simulink model "sim_nomal_regulator"  (R2019a)
settings: Solver=FixedStepAuto  StartTime=0.0  StopTime=20  FixedStep=sT  RelTol=1e-3
InitFcn:
  | sim_param;
values from neighbouring files (symbols this model uses):
  bn = 50    [robot_param.m]    (also in sim_robot_param.m)
  bt = 50    [robot_param.m]    (also in sim_robot_param.m)
  foot_x = 0.07    [robot_param.m]    (also in sim_robot_param.m)
  foot_y = 0.045    [robot_param.m]    (also in sim_robot_param.m)
  foot_z = 0.01    [robot_param.m]    (also in sim_robot_param.m)
  height_plane = 0.025    [robot_param.m]    (also in sim_robot_param.m)
  inix = [0.00 0.00]'    [param.m]    (also in sim_param.m)
  iniXzmax = 0.05    [param.m]    (also in sim_param.m)
  iniXzmin = -0.05    [param.m]    (also in sim_param.m)
  iniy = [0.00 0.00]'    [param.m]    (also in sim_param.m)
  iniYzmax = 0.0625    [param.m]    (also in sim_param.m)
  iniYzmin = -0.0625    [param.m]    (also in sim_param.m)
  kn = 5000    [robot_param.m]    (also in sim_robot_param.m)
  kt = 5000    [robot_param.m]    (also in sim_robot_param.m)
  mu_d = 0.8    [robot_param.m]    (also in sim_robot_param.m)
  mu_s = 2    [robot_param.m]    (also in sim_robot_param.m)
  plane_x = 3    [robot_param.m]    (also in sim_robot_param.m = 6)
  plane_y = 1    [robot_param.m]    (also in sim_robot_param.m)
  R = 20    [param.m]    (also in sim_param.m = 1)
  sT = 0.02    [param.m]    (also in sim_param.m = 0.001)
  torso_offset_x = 0.0    (= 0)    [robot_param.m]    (also in sim_robot_param.m)
  torso_offset_z = -torso_z/2    (= -0.05)    [robot_param.m]    (also in sim_robot_param.m)
  torso_x = 0.1    [robot_param.m]    (also in sim_robot_param.m)
  torso_y = 0.08    [robot_param.m]    (also in sim_robot_param.m)
  torso_z = 0.10    (= 0.1)    [robot_param.m]    (also in sim_robot_param.m)
  w = sqrt(g/zc)    [param.m]    (also in sim_param.m)
  zvt = 1e-3    (= 0.001)    [robot_param.m]    (also in sim_robot_param.m)
undefined symbols (not defined in the file or in its folder): Ad, Bd, Cd, Dd, DiscIntNeverNeededParam, Discrete, sigbuilder_block, Time, X, Y, Z
libraries: nesl_utility x142, sm_lib x86, cstblocks x11, ctrlSharedLib x8
(part 1 of 6)
settings Model: Creator=hideaki  LastModifiedBy=hideaki

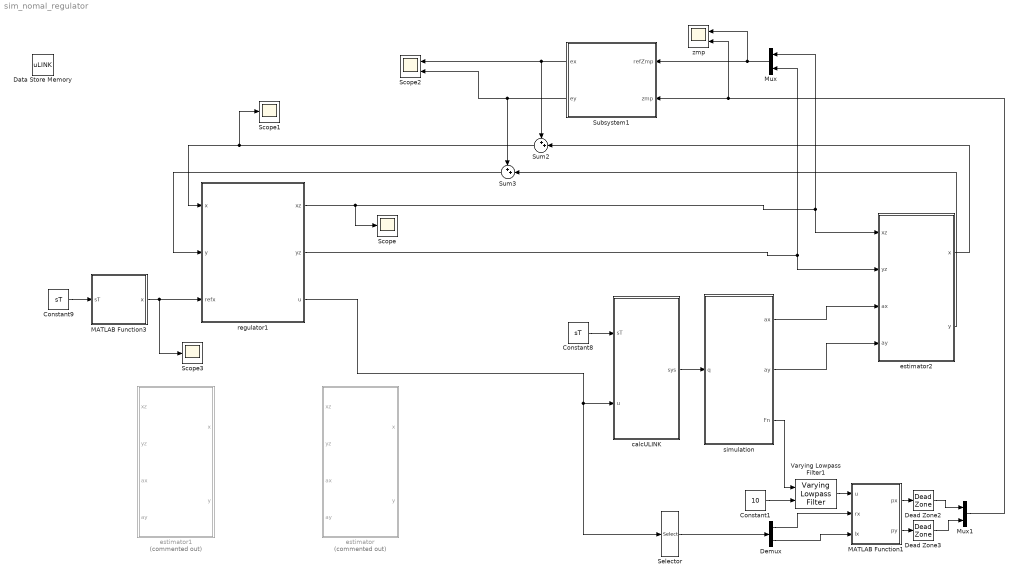
== system sim_nomal_regulator ==
  Constant1 : Constant  Value=10
  Constant8 : Constant  Value=sT
  Constant9 : Constant  Value=sT
  Data Store Memory : DataStoreMemory  DataStoreName=uLINK  ReadBeforeWriteMsg=warning  WriteAfterWriteMsg=warning  WriteAfterReadMsg=warning  InitialValue=uLINK  ShowAdditionalParam=off  OutDataTypeStr=Bus: ULINK  Dimensions=[15 1]
  Dead Zone2 : DeadZone  LowerValue=-1e-5  UpperValue=1e-5  SaturateOnIntegerOverflow=on
  Dead Zone3 : DeadZone  LowerValue=-1e-5  UpperValue=1e-5  SaturateOnIntegerOverflow=on
  Demux : Demux  Outputs=2
  MATLAB Function1 : MATLAB Function  TreatAsAtomicUnit=on
  MATLAB Function3 : MATLAB Function  TreatAsAtomicUnit=on  SystemSampleTime=sT
  Mux : Mux  Inputs=2
  Mux1 : Mux  Inputs=2
  Scope : Scope
  Scope1 : Scope
  Scope2 : Scope  NumInputPorts=2
  Scope3 : Scope
  Selector : Selector  InputPortWidth=8  IndexOptions=Index vector (dialog)  Indices=[3 6]  OutputSizes=1
  Subsystem1 : Subsystem
  Sum2 : Sum  Inputs=++|
  Sum3 : Sum  Inputs=++|
  Varying Lowpass Filter1 : cstblocks/Linear Parameter Varying/Varying Lowpass Filter  N=1
      settings: SourceProductName=Control System Toolbox
  calcULINK : MATLAB Function  TreatAsAtomicUnit=on
  estimator : Subsystem  Commented=on
  estimator1 : Subsystem  Commented=on
  estimator2 : Subsystem
  regulator1 : Subsystem
  simulation : Subsystem
  zmp : Scope  NumInputPorts=2
  wires:
  Constant8/1 -> calcULINK/1(sT)
  calcULINK/1(sys) -> simulation/1(q)
  Constant9/1 -> MATLAB Function3/1(sT)
  simulation/1(ax) -> estimator2/3(ax)
  simulation/2(ay) -> estimator2/4(ay)
  estimator2/2(y) -> Sum3/2
  MATLAB Function3/1(x) -> Scope3/1, regulator1/3(refx)
  regulator1/1(xz) -> Scope/1, estimator2/1(xz), Mux/1
  regulator1/2(yz) -> estimator2/2(yz), Mux/2
  estimator2/1(x) -> Sum2/2
  Varying Lowpass Filter1/1 -> MATLAB Function1/1(u)
  Constant1/1 -> Varying Lowpass Filter1/2
  MATLAB Function1/1(px) -> Dead Zone2/1
  Selector/1 -> Demux/1
  simulation/3(Fn) -> Varying Lowpass Filter1/1
  Demux/1 -> MATLAB Function1/2(rx)
  regulator1/3(u) -> Selector/1, calcULINK/2(u)
  Demux/2 -> MATLAB Function1/3(lx)
  MATLAB Function1/2(py) -> Dead Zone3/1
  Dead Zone2/1 -> Mux1/1
  Dead Zone3/1 -> Mux1/2
  Mux/1 -> zmp/1, Subsystem1/1(refZmp)
  Mux1/1 -> zmp/2, Subsystem1/2(zmp)
  Subsystem1/1(ex) -> Sum2/1, Scope2/1
  Subsystem1/2(ey) -> Sum3/1, Scope2/2
  Sum3/1 -> regulator1/2(y)
  Sum2/1 -> Scope1/1, regulator1/1(x)

== system sim_nomal_regulator/Subsystem1 ==
  note: alphaを外すとおかしくなる
  refZmp : Inport
  zmp : Inport  Port=2
  Demux : Demux  Outputs=2
  Demux2 : Demux  Outputs=2
  Discrete-Time Integrator : DiscreteIntegrator  gainval=1.6  SampleTime=-1  ICPrevOutput=DiscIntNeverNeededParam  ICPrevScaledInput=DiscIntNeverNeededParam
  Discrete-Time Integrator1 : DiscreteIntegrator  SampleTime=-1  ICPrevOutput=DiscIntNeverNeededParam  ICPrevScaledInput=DiscIntNeverNeededParam
  Discrete-Time Integrator2 : DiscreteIntegrator  gainval=1.6  SampleTime=-1  ICPrevOutput=DiscIntNeverNeededParam  ICPrevScaledInput=DiscIntNeverNeededParam
  Discrete-Time Integrator3 : DiscreteIntegrator  SampleTime=-1  ICPrevOutput=DiscIntNeverNeededParam  ICPrevScaledInput=DiscIntNeverNeededParam
  Gain2 : Gain  Gain=0.1
  Gain4 : Gain  Gain=25
  Mux3 : Mux  Inputs=2
  Mux4 : Mux  Inputs=2
  Sum : Sum  Inputs=|-+
  Sum1 : Sum  Inputs=|-+
  Sum3 : Sum  Inputs=+-|
  Sum4 : Sum  Inputs=+-|
  alphax : Constant  Value=0
  alphay : Constant  Value=0
  ex : Outport
  ey : Outport  Port=2
  wires:
  Gain4/1 -> Sum/1
  Demux2/1 -> Sum3/1
  Discrete-Time Integrator2/1 -> Discrete-Time Integrator3/1, Mux4/2
  Demux/1 -> Sum3/2
  Discrete-Time Integrator3/1 -> Mux4/1
  Mux3/1 -> ex/1
  Discrete-Time Integrator1/1 -> Mux3/1
  Demux2/2 -> Sum4/1
  Gain2/1 -> Sum1/1
  Discrete-Time Integrator/1 -> Mux3/2, Discrete-Time Integrator1/1
  Mux4/1 -> ey/1
  Demux/2 -> Sum4/2
  Sum3/1 -> Gain2/1
  zmp/1 -> Demux/1
  Sum4/1 -> Gain4/1
  refZmp/1 -> Demux2/1
  Sum/1 -> Discrete-Time Integrator2/1
  alphay/1 -> Sum/2
  alphax/1 -> Sum1/2
  Sum1/1 -> Discrete-Time Integrator/1

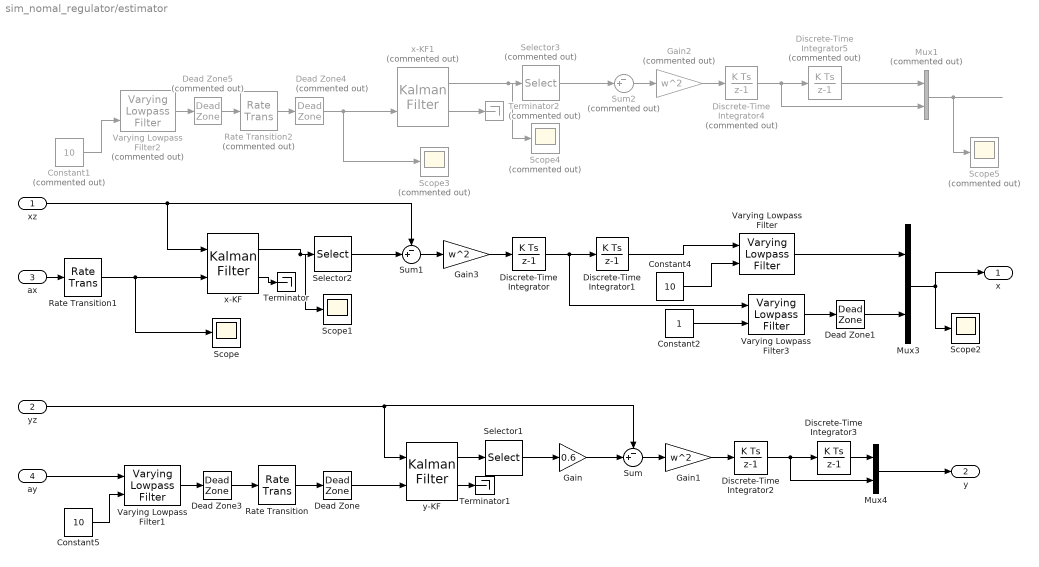
== system sim_nomal_regulator/estimator ==
  xz : Inport
  yz : Inport  Port=2
  ax : Inport  Port=3
  ay : Inport  Port=4
  Constant1 : Constant  Commented=on  Value=10
  Constant2 : Constant
  Constant4 : Constant  Value=10
  Constant5 : Constant  Value=10
  Dead Zone : DeadZone  LowerValue=-1e-3  UpperValue=1e-3  SaturateOnIntegerOverflow=on
  Dead Zone1 : DeadZone  LowerValue=-5e-2  UpperValue=5e-2  SaturateOnIntegerOverflow=on
  Dead Zone3 : DeadZone  LowerValue=-5e-2  UpperValue=5e-2  SaturateOnIntegerOverflow=on
  Dead Zone4 : DeadZone  Commented=on  LowerValue=-1e-3  UpperValue=1e-3  SaturateOnIntegerOverflow=on
  Dead Zone5 : DeadZone  Commented=on  LowerValue=-5e-2  UpperValue=5e-2  SaturateOnIntegerOverflow=on
  Discrete-Time Integrator : DiscreteIntegrator  gainval=1.6  SampleTime=-1  ICPrevOutput=DiscIntNeverNeededParam  ICPrevScaledInput=DiscIntNeverNeededParam
  Discrete-Time Integrator1 : DiscreteIntegrator  SampleTime=-1  ICPrevOutput=DiscIntNeverNeededParam  ICPrevScaledInput=DiscIntNeverNeededParam
  Discrete-Time Integrator2 : DiscreteIntegrator  SampleTime=-1  ICPrevOutput=DiscIntNeverNeededParam  ICPrevScaledInput=DiscIntNeverNeededParam
  Discrete-Time Integrator3 : DiscreteIntegrator  SampleTime=-1  ICPrevOutput=DiscIntNeverNeededParam  ICPrevScaledInput=DiscIntNeverNeededParam
  Discrete-Time Integrator4 : DiscreteIntegrator  Commented=on  gainval=1.6  SampleTime=-1  ICPrevOutput=DiscIntNeverNeededParam  ICPrevScaledInput=DiscIntNeverNeededParam
  Discrete-Time Integrator5 : DiscreteIntegrator  Commented=on  SampleTime=-1  ICPrevOutput=DiscIntNeverNeededParam  ICPrevScaledInput=DiscIntNeverNeededParam
  Gain : Gain  Gain=0.6
  Gain1 : Gain  Gain=w^2
  Gain2 : Gain  Commented=on  Gain=w^2
  Gain3 : Gain  Gain=w^2
  Mux1 : Mux  Commented=on  Inputs=2
  Mux3 : Mux  Inputs=2
  Mux4 : Mux  Inputs=2
  Rate Transition : RateTransition  OutPortSampleTime=sT
  Rate Transition1 : RateTransition  OutPortSampleTime=sT
  Rate Transition2 : RateTransition  Commented=on  OutPortSampleTime=sT
  Scope : Scope
  Scope1 : Scope
  Scope2 : Scope
  Scope3 : Scope  Commented=on
  Scope4 : Scope  Commented=on
  Scope5 : Scope  Commented=on
  Selector1 : Selector  InputPortWidth=2  IndexOptions=Index vector (dialog)  Indices=[1]  OutputSizes=1
  Selector2 : Selector  InputPortWidth=2  IndexOptions=Index vector (dialog)  Indices=[1]  OutputSizes=1
  Selector3 : Selector  Commented=on  InputPortWidth=2  IndexOptions=Index vector (dialog)  Indices=[1]  OutputSizes=1
  Sum : Sum  Inputs=-+|
  Sum1 : Sum  Inputs=-+|
  Sum2 : Sum  Commented=on  Inputs=-+|
  Terminator : Terminator
  Terminator1 : Terminator
  Terminator2 : Terminator  Commented=on
  Varying Lowpass Filter : cstblocks/Linear Parameter Varying/Varying Lowpass Filter  N=1
      settings: SourceProductName=Control System Toolbox
  Varying Lowpass Filter1 : cstblocks/Linear Parameter Varying/Varying Lowpass Filter  N=1
      settings: SourceProductName=Control System Toolbox
  Varying Lowpass Filter2 : cstblocks/Linear Parameter Varying/Varying Lowpass Filter  Commented=on  N=1
      settings: SourceProductName=Control System Toolbox
  Varying Lowpass Filter3 : cstblocks/Linear Parameter Varying/Varying Lowpass Filter  N=1
      settings: SourceProductName=Control System Toolbox
  x-KF : ctrlSharedLib/Kalman Filter  TimeDomain=Discrete-Time  UseCurrentEstimator=on  ModelSource=Individual A, B, C, D matrices  ModelSourceVariable=ss(0.95,1,1,0,1)  A=Ad  B=Bd  C=Cd  D=Dd  NumberOfStates=1  NumberOfInputs=1  NumberOfOutputs=1  InitialEstimateSource=Dialog  X0=inix  P0=[100 50]'  UseK=off  UseGH=off  NumberOfProcessNoiseInputs=1  G=[0 0]'  TimeInvariantG=on  H=10  TimeInvariantH=on  Q=Q  TimeInvariantQ=on  R=R  TimeInvariantR=on  N=0  TimeInvariantN=on  AddInputPort=on  AddEnablePort=off  OutputEstimatedY=on  OutputP=off  Ts=sT
      settings: SourceProductBaseCode=CT
  x-KF1 : ctrlSharedLib/Kalman Filter  Commented=on  TimeDomain=Discrete-Time  UseCurrentEstimator=on  ModelSource=Individual A, B, C, D matrices  ModelSourceVariable=ss(0.95,1,1,0,1)  A=Ad  B=Bd  C=Cd  D=Dd  NumberOfStates=1  NumberOfInputs=1  NumberOfOutputs=1  InitialEstimateSource=Dialog  X0=inix  P0=[100 50]'  UseK=off  UseGH=off  NumberOfProcessNoiseInputs=1  G=[0 0]'  TimeInvariantG=on  H=10  TimeInvariantH=on  Q=Q  TimeInvariantQ=on  R=R  TimeInvariantR=on  N=0  TimeInvariantN=on  AddInputPort=on  AddEnablePort=off  OutputEstimatedY=on  OutputP=off  Ts=sT
      settings: SourceProductBaseCode=CT
  y-KF : ctrlSharedLib/Kalman Filter  TimeDomain=Discrete-Time  UseCurrentEstimator=on  ModelSource=Individual A, B, C, D matrices  ModelSourceVariable=ss(0.95,1,1,0,1)  A=Ad  B=Bd  C=Cd  D=Dd  NumberOfStates=1  NumberOfInputs=1  NumberOfOutputs=1  InitialEstimateSource=Dialog  X0=iniy  P0=10  UseK=off  UseGH=off  NumberOfProcessNoiseInputs=1  G=[0 0]'  TimeInvariantG=on  H=10  TimeInvariantH=on  Q=Q  TimeInvariantQ=on  R=R  TimeInvariantR=on  N=0  TimeInvariantN=on  AddInputPort=on  AddEnablePort=off  OutputEstimatedY=on  OutputP=off  Ts=sT
      settings: SourceProductBaseCode=CT
  x : Outport
  y : Outport  Port=2
  wires:
  Sum/1 -> Gain1/1
  Dead Zone/1 -> y-KF/2
  Selector1/1 -> Gain/1
  Discrete-Time Integrator2/1 -> Discrete-Time Integrator3/1, Mux4/2
  Sum1/1 -> Gain3/1
  Discrete-Time Integrator3/1 -> Mux4/1
  Discrete-Time Integrator/1 -> Varying Lowpass Filter3/1, Discrete-Time Integrator1/1
  Gain3/1 -> Discrete-Time Integrator/1
  y-KF/2 -> Terminator1/1
  Gain1/1 -> Discrete-Time Integrator2/1
  Varying Lowpass Filter1/1 -> Dead Zone3/1
  xz/1 -> Sum1/1, x-KF/1
  Rate Transition/1 -> Dead Zone/1
  y-KF/1 -> Selector1/1
  Constant4/1 -> Varying Lowpass Filter/2
  Constant5/1 -> Varying Lowpass Filter1/2
  Varying Lowpass Filter/1 -> Mux3/1
  x-KF/1 -> Scope1/1, Selector2/1
  yz/1 -> y-KF/1, Sum/1
  Discrete-Time Integrator1/1 -> Varying Lowpass Filter/1
  Gain/1 -> Sum/2
  Selector2/1 -> Sum1/2
  Mux3/1 -> Scope2/1, x/1
  Mux4/1 -> y/1
  x-KF/2 -> Terminator/1
  ay/1 -> Varying Lowpass Filter1/1
  ax/1 -> Rate Transition1/1
  Dead Zone3/1 -> Rate Transition/1
  Dead Zone5/1 -> Rate Transition2/1
  Dead Zone4/1 -> Scope3/1, x-KF1/2
  Rate Transition2/1 -> Dead Zone4/1
  x-KF1/2 -> Terminator2/1
  Selector3/1 -> Sum2/2
  Mux1/1 -> Scope5/1
  x-KF1/1 -> Scope4/1, Selector3/1
  Constant1/1 -> Varying Lowpass Filter2/2
  ? -> Varying Lowpass Filter2/1
  Gain2/1 -> Discrete-Time Integrator4/1
  Discrete-Time Integrator5/1 -> Mux1/1
  ? -> Sum2/1, x-KF1/1
  Varying Lowpass Filter2/1 -> Dead Zone5/1
  Discrete-Time Integrator4/1 -> Discrete-Time Integrator5/1, Mux1/2
  Sum2/1 -> Gain2/1
  Varying Lowpass Filter3/1 -> Dead Zone1/1
  Rate Transition1/1 -> Scope/1, x-KF/2
  Constant2/1 -> Varying Lowpass Filter3/2
  Dead Zone1/1 -> Mux3/2

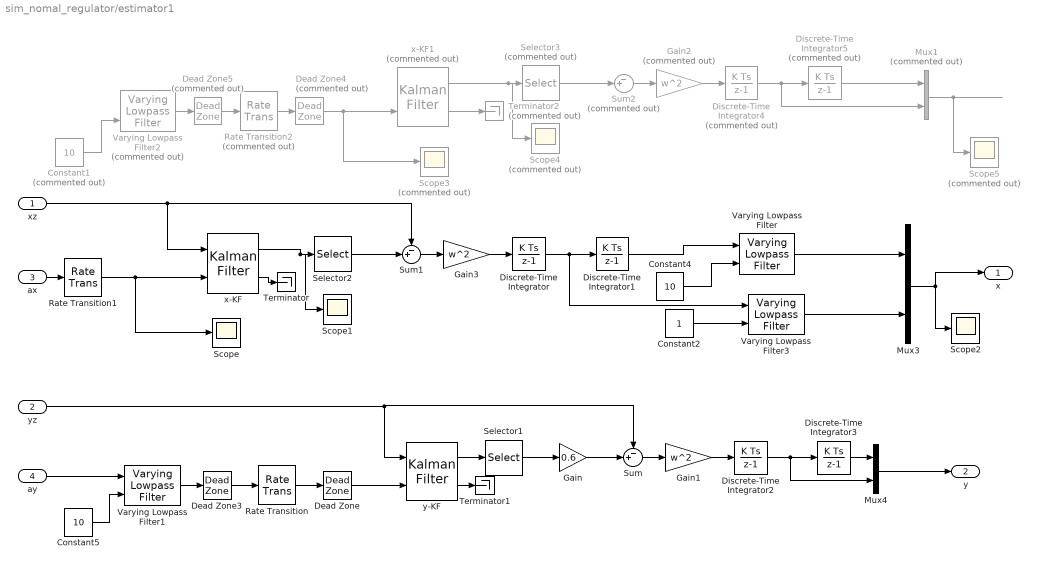
== system sim_nomal_regulator/estimator1 ==
  xz : Inport
  yz : Inport  Port=2
  ax : Inport  Port=3
  ay : Inport  Port=4
  Constant1 : Constant  Commented=on  Value=10
  Constant2 : Constant
  Constant4 : Constant  Value=10
  Constant5 : Constant  Value=10
  Dead Zone : DeadZone  LowerValue=-1e-3  UpperValue=1e-3  SaturateOnIntegerOverflow=on
  Dead Zone3 : DeadZone  LowerValue=-5e-2  UpperValue=5e-2  SaturateOnIntegerOverflow=on
  Dead Zone4 : DeadZone  Commented=on  LowerValue=-1e-3  UpperValue=1e-3  SaturateOnIntegerOverflow=on
  Dead Zone5 : DeadZone  Commented=on  LowerValue=-5e-2  UpperValue=5e-2  SaturateOnIntegerOverflow=on
  Discrete-Time Integrator : DiscreteIntegrator  gainval=1.6  SampleTime=-1  ICPrevOutput=DiscIntNeverNeededParam  ICPrevScaledInput=DiscIntNeverNeededParam
  Discrete-Time Integrator1 : DiscreteIntegrator  SampleTime=-1  ICPrevOutput=DiscIntNeverNeededParam  ICPrevScaledInput=DiscIntNeverNeededParam
  Discrete-Time Integrator2 : DiscreteIntegrator  SampleTime=-1  ICPrevOutput=DiscIntNeverNeededParam  ICPrevScaledInput=DiscIntNeverNeededParam
  Discrete-Time Integrator3 : DiscreteIntegrator  SampleTime=-1  ICPrevOutput=DiscIntNeverNeededParam  ICPrevScaledInput=DiscIntNeverNeededParam
  Discrete-Time Integrator4 : DiscreteIntegrator  Commented=on  gainval=1.6  SampleTime=-1  ICPrevOutput=DiscIntNeverNeededParam  ICPrevScaledInput=DiscIntNeverNeededParam
  Discrete-Time Integrator5 : DiscreteIntegrator  Commented=on  SampleTime=-1  ICPrevOutput=DiscIntNeverNeededParam  ICPrevScaledInput=DiscIntNeverNeededParam
  Gain : Gain  Gain=0.6
  Gain1 : Gain  Gain=w^2
  Gain2 : Gain  Commented=on  Gain=w^2
  Gain3 : Gain  Gain=w^2
  Mux1 : Mux  Commented=on  Inputs=2
  Mux3 : Mux  Inputs=2
  Mux4 : Mux  Inputs=2
  Rate Transition : RateTransition  OutPortSampleTime=sT
  Rate Transition1 : RateTransition  OutPortSampleTime=sT
  Rate Transition2 : RateTransition  Commented=on  OutPortSampleTime=sT
  Scope : Scope
  Scope1 : Scope
  Scope2 : Scope
  Scope3 : Scope  Commented=on
  Scope4 : Scope  Commented=on
  Scope5 : Scope  Commented=on
  Selector1 : Selector  InputPortWidth=2  IndexOptions=Index vector (dialog)  Indices=[1]  OutputSizes=1
  Selector2 : Selector  InputPortWidth=2  IndexOptions=Index vector (dialog)  Indices=[1]  OutputSizes=1
  Selector3 : Selector  Commented=on  InputPortWidth=2  IndexOptions=Index vector (dialog)  Indices=[1]  OutputSizes=1
  Sum : Sum  Inputs=-+|
  Sum1 : Sum  Inputs=-+|
  Sum2 : Sum  Commented=on  Inputs=-+|
  Terminator : Terminator
  Terminator1 : Terminator
  Terminator2 : Terminator  Commented=on
  Varying Lowpass Filter : cstblocks/Linear Parameter Varying/Varying Lowpass Filter  N=1
      settings: SourceProductName=Control System Toolbox
  Varying Lowpass Filter1 : cstblocks/Linear Parameter Varying/Varying Lowpass Filter  N=1
      settings: SourceProductName=Control System Toolbox
  Varying Lowpass Filter2 : cstblocks/Linear Parameter Varying/Varying Lowpass Filter  Commented=on  N=1
      settings: SourceProductName=Control System Toolbox
  Varying Lowpass Filter3 : cstblocks/Linear Parameter Varying/Varying Lowpass Filter  N=1
      settings: SourceProductName=Control System Toolbox
  x-KF : ctrlSharedLib/Kalman Filter  TimeDomain=Discrete-Time  UseCurrentEstimator=on  ModelSource=Individual A, B, C, D matrices  ModelSourceVariable=ss(0.95,1,1,0,1)  A=Ad  B=Bd  C=Cd  D=Dd  NumberOfStates=1  NumberOfInputs=1  NumberOfOutputs=1  InitialEstimateSource=Dialog  X0=inix  P0=[100 50]'  UseK=off  UseGH=off  NumberOfProcessNoiseInputs=1  G=[0 0]'  TimeInvariantG=on  H=10  TimeInvariantH=on  Q=Q  TimeInvariantQ=on  R=R  TimeInvariantR=on  N=0  TimeInvariantN=on  AddInputPort=on  AddEnablePort=off  OutputEstimatedY=on  OutputP=off  Ts=sT
      settings: SourceProductBaseCode=CT
  x-KF1 : ctrlSharedLib/Kalman Filter  Commented=on  TimeDomain=Discrete-Time  UseCurrentEstimator=on  ModelSource=Individual A, B, C, D matrices  ModelSourceVariable=ss(0.95,1,1,0,1)  A=Ad  B=Bd  C=Cd  D=Dd  NumberOfStates=1  NumberOfInputs=1  NumberOfOutputs=1  InitialEstimateSource=Dialog  X0=inix  P0=[100 50]'  UseK=off  UseGH=off  NumberOfProcessNoiseInputs=1  G=[0 0]'  TimeInvariantG=on  H=10  TimeInvariantH=on  Q=Q  TimeInvariantQ=on  R=R  TimeInvariantR=on  N=0  TimeInvariantN=on  AddInputPort=on  AddEnablePort=off  OutputEstimatedY=on  OutputP=off  Ts=sT
      settings: SourceProductBaseCode=CT
  y-KF : ctrlSharedLib/Kalman Filter  TimeDomain=Discrete-Time  UseCurrentEstimator=on  ModelSource=Individual A, B, C, D matrices  ModelSourceVariable=ss(0.95,1,1,0,1)  A=Ad  B=Bd  C=Cd  D=Dd  NumberOfStates=1  NumberOfInputs=1  NumberOfOutputs=1  InitialEstimateSource=Dialog  X0=iniy  P0=10  UseK=off  UseGH=off  NumberOfProcessNoiseInputs=1  G=[0 0]'  TimeInvariantG=on  H=10  TimeInvariantH=on  Q=Q  TimeInvariantQ=on  R=R  TimeInvariantR=on  N=0  TimeInvariantN=on  AddInputPort=on  AddEnablePort=off  OutputEstimatedY=on  OutputP=off  Ts=sT
      settings: SourceProductBaseCode=CT
  x : Outport
  y : Outport  Port=2
  wires:
  Sum/1 -> Gain1/1
  Dead Zone/1 -> y-KF/2
  Selector1/1 -> Gain/1
  Discrete-Time Integrator2/1 -> Discrete-Time Integrator3/1, Mux4/2
  Sum1/1 -> Gain3/1
  Discrete-Time Integrator3/1 -> Mux4/1
  Discrete-Time Integrator/1 -> Varying Lowpass Filter3/1, Discrete-Time Integrator1/1
  Gain3/1 -> Discrete-Time Integrator/1
  y-KF/2 -> Terminator1/1
  Gain1/1 -> Discrete-Time Integrator2/1
  Varying Lowpass Filter1/1 -> Dead Zone3/1
  xz/1 -> Sum1/1, x-KF/1
  Rate Transition/1 -> Dead Zone/1
  y-KF/1 -> Selector1/1
  Constant4/1 -> Varying Lowpass Filter/2
  Constant5/1 -> Varying Lowpass Filter1/2
  Varying Lowpass Filter/1 -> Mux3/1
  x-KF/1 -> Scope1/1, Selector2/1
  yz/1 -> y-KF/1, Sum/1
  Discrete-Time Integrator1/1 -> Varying Lowpass Filter/1
  Gain/1 -> Sum/2
  Selector2/1 -> Sum1/2
  Mux3/1 -> Scope2/1, x/1
  Mux4/1 -> y/1
  x-KF/2 -> Terminator/1
  ay/1 -> Varying Lowpass Filter1/1
  ax/1 -> Rate Transition1/1
  Dead Zone3/1 -> Rate Transition/1
  Dead Zone5/1 -> Rate Transition2/1
  Dead Zone4/1 -> Scope3/1, x-KF1/2
  Rate Transition2/1 -> Dead Zone4/1
  x-KF1/2 -> Terminator2/1
  Selector3/1 -> Sum2/2
  Mux1/1 -> Scope5/1
  x-KF1/1 -> Scope4/1, Selector3/1
  Constant1/1 -> Varying Lowpass Filter2/2
  ? -> Varying Lowpass Filter2/1
  Gain2/1 -> Discrete-Time Integrator4/1
  Discrete-Time Integrator5/1 -> Mux1/1
  ? -> Sum2/1, x-KF1/1
  Varying Lowpass Filter2/1 -> Dead Zone5/1
  Discrete-Time Integrator4/1 -> Discrete-Time Integrator5/1, Mux1/2
  Sum2/1 -> Gain2/1
  Varying Lowpass Filter3/1 -> Mux3/2
  Rate Transition1/1 -> Scope/1, x-KF/2
  Constant2/1 -> Varying Lowpass Filter3/2

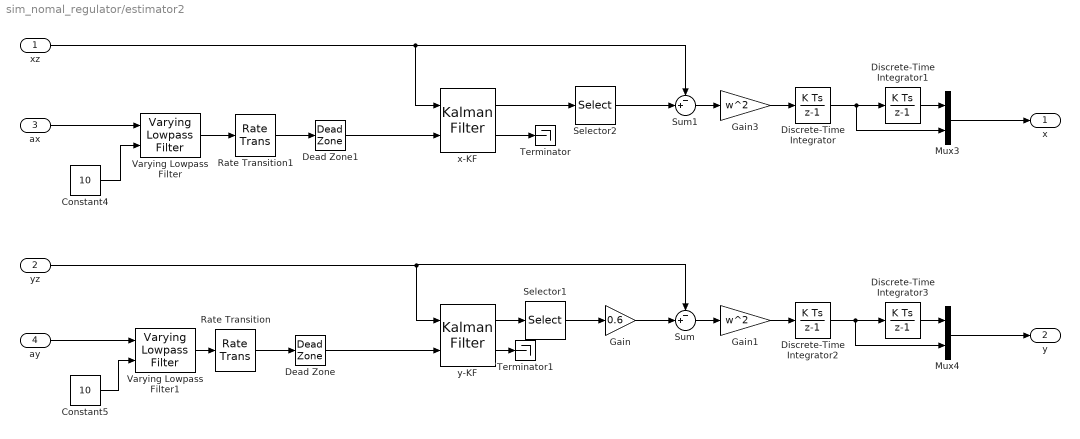
== system sim_nomal_regulator/estimator2 ==
  xz : Inport
  yz : Inport  Port=2
  ax : Inport  Port=3
  ay : Inport  Port=4
  Constant4 : Constant  Value=10
  Constant5 : Constant  Value=10
  Dead Zone : DeadZone  LowerValue=-1e-3  UpperValue=1e-3  SaturateOnIntegerOverflow=on
  Dead Zone1 : DeadZone  LowerValue=-1e-3  UpperValue=1e-3  SaturateOnIntegerOverflow=on
  Discrete-Time Integrator : DiscreteIntegrator  gainval=1.6  SampleTime=-1  ICPrevOutput=DiscIntNeverNeededParam  ICPrevScaledInput=DiscIntNeverNeededParam
  Discrete-Time Integrator1 : DiscreteIntegrator  SampleTime=-1  ICPrevOutput=DiscIntNeverNeededParam  ICPrevScaledInput=DiscIntNeverNeededParam
  Discrete-Time Integrator2 : DiscreteIntegrator  SampleTime=-1  ICPrevOutput=DiscIntNeverNeededParam  ICPrevScaledInput=DiscIntNeverNeededParam
  Discrete-Time Integrator3 : DiscreteIntegrator  SampleTime=-1  ICPrevOutput=DiscIntNeverNeededParam  ICPrevScaledInput=DiscIntNeverNeededParam
  Gain : Gain  Gain=0.6
  Gain1 : Gain  Gain=w^2
  Gain3 : Gain  Gain=w^2
  Mux3 : Mux  Inputs=2
  Mux4 : Mux  Inputs=2
  Rate Transition : RateTransition  OutPortSampleTime=sT
  Rate Transition1 : RateTransition  OutPortSampleTime=sT
  Selector1 : Selector  InputPortWidth=2  IndexOptions=Index vector (dialog)  Indices=[1]  OutputSizes=1
  Selector2 : Selector  InputPortWidth=2  IndexOptions=Index vector (dialog)  Indices=[1]  OutputSizes=1
  Sum : Sum  Inputs=-+|
  Sum1 : Sum  Inputs=-+|
  Terminator : Terminator
  Terminator1 : Terminator
  Varying Lowpass Filter : cstblocks/Linear Parameter Varying/Varying Lowpass Filter  N=1
      settings: SourceProductName=Control System Toolbox
  Varying Lowpass Filter1 : cstblocks/Linear Parameter Varying/Varying Lowpass Filter  N=1
      settings: SourceProductName=Control System Toolbox
  x-KF : ctrlSharedLib/Kalman Filter  TimeDomain=Discrete-Time  UseCurrentEstimator=on  ModelSource=Individual A, B, C, D matrices  ModelSourceVariable=ss(0.95,1,1,0,1)  A=Ad  B=Bd  C=Cd  D=Dd  NumberOfStates=1  NumberOfInputs=1  NumberOfOutputs=1  InitialEstimateSource=Dialog  X0=inix  P0=[100 50]'  UseK=off  UseGH=off  NumberOfProcessNoiseInputs=1  G=[0 0]'  TimeInvariantG=on  H=10  TimeInvariantH=on  Q=Q  TimeInvariantQ=on  R=R  TimeInvariantR=on  N=0  TimeInvariantN=on  AddInputPort=on  AddEnablePort=off  OutputEstimatedY=on  OutputP=off  Ts=sT
      settings: SourceProductBaseCode=CT
  y-KF : ctrlSharedLib/Kalman Filter  TimeDomain=Discrete-Time  UseCurrentEstimator=on  ModelSource=Individual A, B, C, D matrices  ModelSourceVariable=ss(0.95,1,1,0,1)  A=Ad  B=Bd  C=Cd  D=Dd  NumberOfStates=1  NumberOfInputs=1  NumberOfOutputs=1  InitialEstimateSource=Dialog  X0=iniy  P0=10  UseK=off  UseGH=off  NumberOfProcessNoiseInputs=1  G=[0 0]'  TimeInvariantG=on  H=10  TimeInvariantH=on  Q=Q  TimeInvariantQ=on  R=R  TimeInvariantR=on  N=0  TimeInvariantN=on  AddInputPort=on  AddEnablePort=off  OutputEstimatedY=on  OutputP=off  Ts=sT
      settings: SourceProductBaseCode=CT
  x : Outport
  y : Outport  Port=2
  wires:
  Sum/1 -> Gain1/1
  Dead Zone/1 -> y-KF/2
  Selector1/1 -> Gain/1
  Discrete-Time Integrator2/1 -> Discrete-Time Integrator3/1, Mux4/2
  Rate Transition1/1 -> Dead Zone1/1
  Sum1/1 -> Gain3/1
  Discrete-Time Integrator3/1 -> Mux4/1
  Discrete-Time Integrator/1 -> Discrete-Time Integrator1/1, Mux3/2
  ax/1 -> Varying Lowpass Filter/1
  Gain3/1 -> Discrete-Time Integrator/1
  y-KF/2 -> Terminator1/1
  Dead Zone1/1 -> x-KF/2
  Gain1/1 -> Discrete-Time Integrator2/1
  Varying Lowpass Filter1/1 -> Rate Transition/1
  xz/1 -> Sum1/1, x-KF/1
  Rate Transition/1 -> Dead Zone/1
  y-KF/1 -> Selector1/1
  Constant4/1 -> Varying Lowpass Filter/2
  Constant5/1 -> Varying Lowpass Filter1/2
  Varying Lowpass Filter/1 -> Rate Transition1/1
  x-KF/1 -> Selector2/1
  yz/1 -> y-KF/1, Sum/1
  Discrete-Time Integrator1/1 -> Mux3/1
  Gain/1 -> Sum/2
  Selector2/1 -> Sum1/2
  Mux3/1 -> x/1
  Mux4/1 -> y/1
  x-KF/2 -> Terminator/1
  ay/1 -> Varying Lowpass Filter1/1

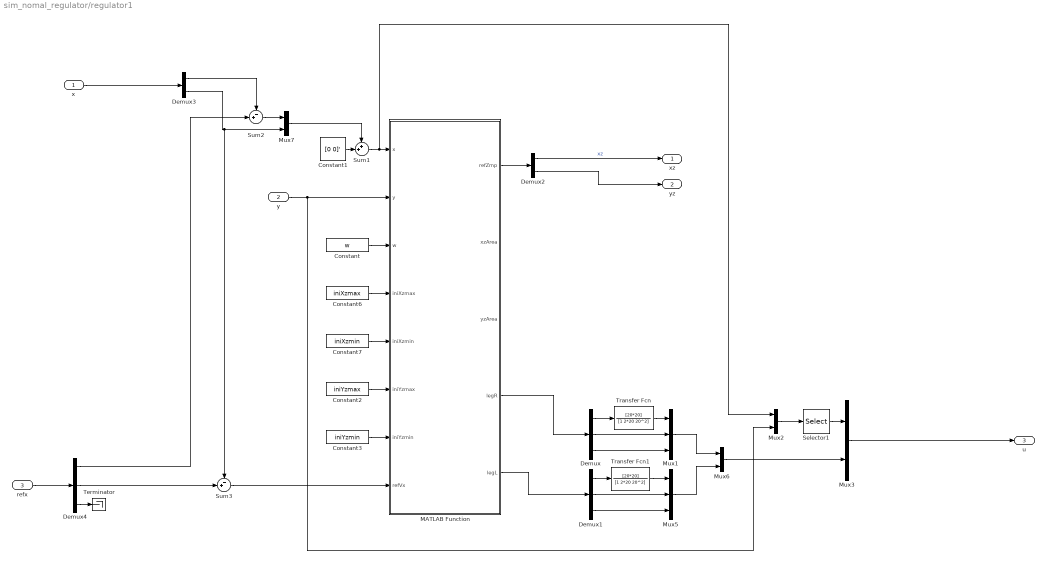
== system sim_nomal_regulator/regulator1 ==
  x : Inport
  y : Inport  Port=2
  refx : Inport  Port=3
  Constant : Constant  Value=w
  Constant1 : Constant  Value=[0 0]'
  Constant2 : Constant  Value=iniYzmax
  Constant3 : Constant  Value=iniYzmin
  Constant6 : Constant  Value=iniXzmax
  Constant7 : Constant  Value=iniXzmin
  Demux : Demux  Outputs=3
  Demux1 : Demux  Outputs=3
  Demux2 : Demux  Outputs=2
  Demux3 : Demux  Outputs=2
  Demux4 : Demux  Outputs=3
  MATLAB Function : MATLAB Function  TreatAsAtomicUnit=on  SystemSampleTime=sT
  Mux1 : Mux  Inputs=3
  Mux{2..3,6..7} (4 alike) : Mux  Inputs=2
  Mux5 : Mux  Inputs=3
  Selector1 : Selector  InputPortWidth=4  IndexOptions=Index vector (dialog)  Indices=[1 3]  OutputSizes=1
  Sum1 : Sum  Inputs=++|
  Sum2 : Sum  Inputs=-+|
  Sum3 : Sum  Inputs=-+|
  Terminator : Terminator
  Transfer Fcn : TransferFcn  Numerator=[20*20]  Denominator=[1 2*20 20^2]
  Transfer Fcn1 : TransferFcn  Numerator=[20*20]  Denominator=[1 2*20 20^2]
  xz : Outport
  yz : Outport  Port=2
  u : Outport  Port=3
  wires:
  Constant/1 -> MATLAB Function/3(w)
  Demux4/2 -> Sum3/2
  MATLAB Function/4(legR) -> Demux/1
  Transfer Fcn1/1 -> Mux5/1
  Constant3/1 -> MATLAB Function/7(iniYzmin)
  MATLAB Function/1(refZmp) -> Demux2/1
  Constant2/1 -> MATLAB Function/6(iniYzmax)
  Transfer Fcn/1 -> Mux1/1
  Demux/3 -> Mux1/3
  Demux3/1 -> Sum2/1
  Demux2/1 -> xz/1  "xz"
  Demux4/1 -> Sum2/2
  x/1 -> Demux3/1
  MATLAB Function/5(legL) -> Demux1/1
  Demux3/2 -> Mux7/2, Sum3/1
  Demux1/2 -> Mux5/2
  Demux/1 -> Transfer Fcn/1
  Demux1/3 -> Mux5/3
  refx/1 -> Demux4/1
  Demux2/2 -> yz/1
  Constant7/1 -> MATLAB Function/5(iniXzmin)
  Demux1/1 -> Transfer Fcn1/1
  Mux5/1 -> Mux6/2
  Constant6/1 -> MATLAB Function/4(iniXzmax)
  Demux/2 -> Mux1/2
  Mux1/1 -> Mux6/1
  Demux4/3 -> Terminator/1
  Constant1/1 -> Sum1/2
  Sum3/1 -> MATLAB Function/8(refVx)
  Sum2/1 -> Mux7/1
  Mux7/1 -> Sum1/1
  Mux3/1 -> u/1
  Selector1/1 -> Mux3/1
  Mux2/1 -> Selector1/1
  Mux6/1 -> Mux3/2
  Sum1/1 -> Mux2/1, MATLAB Function/1(x)
  y/1 -> MATLAB Function/2(y), Mux2/2

== system sim_nomal_regulator/simulation ==
  q : Inport
  6-DOF Joint : sm_lib/Joints/6-DOF Joint  SenseConstraintForce=off  SenseConstraintForceX=off  SenseConstraintForceY=off  SenseConstraintForceZ=off  SenseConstraintTorque=off  SenseConstraintTorqueX=off  SenseConstraintTorqueY=off  SenseConstraintTorqueZ=off  SenseTotalForce=off  SenseTotalForceX=off  SenseTotalForceY=off  SenseTotalForceZ=off  SenseTotalTorque=off  SenseTotalTorqueX=off  SenseTotalTorqueY=off  SenseTotalTorqueZ=off  CompositeWrenchDir=FollowerOnBase  CompositeWrenchFrame=BaseFrame  PxEquilibriumPosition=0  PxEquilibriumPositionUnits=m  PxSpringStiffness=0  PxSpringStiffnessUnits=N/m  PxDampingCoefficient=world_damping  PxDampingCoefficientUnits=N/(m/s)  PxTorqueActuationMode=NoTorque  PxMotionActuationMode=ComputedMotion  PxSensePosition=off  PxSenseVelocity=off  PxSenseAcceleration=off  PxSenseTorqueForce=off  PxSenseLowerLimitTorqueForce=off  PxSenseUpperLimitTorqueForce=off  PxLowerLimitSpecify=off  PxLowerLimitBound=-1  PxLowerLimitBoundUnits=m  PxLowerLimitStiffness=1e6  PxLowerLimitStiffnessUnits=N/m  PxLowerLimitDamping=1e3  PxLowerLimitDampingUnits=N/(m/s)  PxLowerLimitTransitionRegionWidth=1e-4  PxLowerLimitTransitionRegionWidthUnits=m  PxUpperLimitSpecify=off  PxUpperLimitBound=1  PxUpperLimitBoundUnits=m  PxUpperLimitStiffness=1e6  PxUpperLimitStiffnessUnits=N/m  PxUpperLimitDamping=1e3  PxUpperLimitDampingUnits=N/(m/s)  PxUpperLimitTransitionRegionWidth=1e-4  PxUpperLimitTransitionRegionWidthUnits=m  PxPositionTargetSpecify=on  PxPositionTargetPriority=High  PxPositionTargetValue=0  PxPositionTargetValueUnits=m  PxVelocityTargetSpecify=off  PxVelocityTargetPriority=High  PxVelocityTargetValue=0  PxVelocityTargetValueUnits=m/s  PyEquilibriumPosition=0  PyEquilibriumPositionUnits=m  PySpringStiffness=0  PySpringStiffnessUnits=N/m  PyDampingCoefficient=world_damping  PyDampingCoefficientUnits=N/(m/s)  PyTorqueActuationMode=NoTorque  PyMotionActuationMode=ComputedMotion  PySensePosition=off  PySenseVelocity=off  PySenseAcceleration=off  PySenseTorqueForce=off  PySenseLowerLimitTorqueForce=off  PySenseUpperLimitTorqueForce=off  PyLowerLimitSpecify=off  PyLowerLimitBound=-1  PyLowerLimitBoundUnits=m  PyLowerLimitStiffness=1e6  PyLowerLimitStiffnessUnits=N/m  PyLowerLimitDamping=1e3  PyLowerLimitDampingUnits=N/(m/s)  PyLowerLimitTransitionRegionWidth=1e-4  PyLowerLimitTransitionRegionWidthUnits=m  PyUpperLimitSpecify=off  PyUpperLimitBound=1  PyUpperLimitBoundUnits=m  PyUpperLimitStiffness=1e6  PyUpperLimitStiffnessUnits=N/m  PyUpperLimitDamping=1e3  PyUpperLimitDampingUnits=N/(m/s)  PyUpperLimitTransitionRegionWidth=1e-4  PyUpperLimitTransitionRegionWidthUnits=m  PyPositionTargetSpecify=on  PyPositionTargetPriority=High  PyPositionTargetValue=0  PyPositionTargetValueUnits=m  PyVelocityTargetSpecify=off  PyVelocityTargetPriority=High  PyVelocityTargetValue=0  PyVelocityTargetValueUnits=m/s  PzEquilibriumPosition=0  PzEquilibriumPositionUnits=m  PzSpringStiffness=0  PzSpringStiffnessUnits=N/m  PzDampingCoefficient=world_damping  PzDampingCoefficientUnits=N/(m/s)  PzTorqueActuationMode=NoTorque  PzMotionActuationMode=ComputedMotion  PzSensePosition=off  PzSenseVelocity=off  PzSenseAcceleration=off  PzSenseTorqueForce=off  PzSenseLowerLimitTorqueForce=off  PzSenseUpperLimitTorqueForce=off  PzLowerLimitSpecify=off  PzLowerLimitBound=-1  PzLowerLimitBoundUnits=m  PzLowerLimitStiffness=1e6  PzLowerLimitStiffnessUnits=N/m  PzLowerLimitDamping=1e3  PzLowerLimitDampingUnits=N/(m/s)  PzLowerLimitTransitionRegionWidth=1e-4  PzLowerLimitTransitionRegionWidthUnits=m  PzUpperLimitSpecify=off  PzUpperLimitBound=1  PzUpperLimitBoundUnits=m  PzUpperLimitStiffness=1e6  PzUpperLimitStiffnessUnits=N/m  PzUpperLimitDamping=1e3  PzUpperLimitDampingUnits=N/(m/s)  PzUpperLimitTransitionRegionWidth=1e-4  PzUpperLimitTransitionRegionWidthUnits=m  PzPositionTargetSpecify=on  PzPositionTargetPriority=High  PzPositionTargetValue=init_height  PzPositionTargetValueUnits=m  PzVelocityTargetSpecify=off  PzVelocityTargetPriority=High  PzVelocityTargetValue=0  PzVelocityTargetValueUnits=m/s  SphDefPosRotationMethod=None  SphDefPosRotationAngleUnits=deg  SphDefPosRotationStandardAxis=+Z  SphDefPosRotationAngle=0.0  SphDefPosRotationArbitraryAxis=[0 0 1]  SphDefPosFollAlignAxisA=+X  SphDefPosBaseAlignAxisA=+Y  SphDefPosFollAlignAxisB=+Y  SphDefPosBaseAlignAxisB=+Z  SphDefPosRotationSequenceAxes=FollowerAxes  SphDefPosRotationSequence=XYX  SphDefPosRotationSequenceAngles=[0 0 0]  SphDefPosRotationSequenceAnglesUnits=deg  SphDefPosRotationMatrix=[1 0 0; 0 1 0; 0 0 1]  SphEqPosRotationMethod=None  SphEqPosRotationAngleUnits=deg  SphEqPosRotationStandardAxis=+Z  SphEqPosRotationAngle=0.0  SphEqPosRotationArbitraryAxis=[0 0 1]  SphEqPosFollAlignAxisA=+X  SphEqPosBaseAlignAxisA=+Y  SphEqPosFollAlignAxisB=+Y  SphEqPosBaseAlignAxisB=+Z  SphEqPosRotationSequenceAxes=FollowerAxes  SphEqPosRotationSequence=XYX  SphEqPosRotationSequenceAngles=[0 0 0]  SphEqPosRotationSequenceAnglesUnits=deg  SphEqPosRotationMatrix=[1 0 0; 0 1 0; 0 0 1]  SphSpringStiffness=0  SphSpringStiffnessUnits=N*m/deg  SphDampingCoefficient=world_rot_damping  SphDampingCoefficientUnits=N*m/(rad/s)  SphActuateTorqueX=off  SphActuateTorqueY=off  SphActuateTorqueZ=off  SphActuateTorque=off  SphTorqueActuationMode=NoTorque  SphMotionActuationMode=ComputedMotion  SphActuationFrame=BaseFrame  SphSensePosition=off  SphSenseVelocityX=off  SphSenseVelocityY=off  SphSenseVelocityZ=off  SphSenseVelocity=off  SphSenseAccelerationX=off  SphSenseAccelerationY=off  SphSenseAccelerationZ=off  SphSenseAcceleration=off  SphSenseTorqueX=off  SphSenseTorqueY=off  SphSenseTorqueZ=off  SphSenseTorqueForce=off  SphSenseLowerLimitTorqueMag=off  SphSenseUpperLimitTorqueMag=off  SphSensingFrame=BaseFrame  SphLowerLimitSpecify=off  SphLowerLimitBound=15  SphLowerLimitBoundUnits=deg  SphLowerLimitStiffness=1e4  SphLowerLimitStiffnessUnits=N*m/deg  SphLowerLimitDamping=10  SphLowerLimitDampingUnits=N*m/(deg/s)  SphLowerLimitTransitionRegionWidth=0.1  SphLowerLimitTransitionRegionWidthUnits=deg  SphUpperLimitSpecify=off  SphUpperLimitBound=45  SphUpperLimitBoundUnits=deg  SphUpperLimitStiffness=1e4  SphUpperLimitStiffnessUnits=N*m/deg  SphUpperLimitDamping=10  SphUpperLimitDampingUnits=N*m/(deg/s)  SphUpperLimitTransitionRegionWidth=0.1  SphUpperLimitTransitionRegionWidthUnits=deg  SphPositionTargetRotationMethod=None  SphPositionTargetRotationAngleUnits=deg  SphPositionTargetRotationStandardAxis=+Z  SphPositionTargetRotationAngle=0.0  SphPositionTargetRotationArbitraryAxis=[0 0 1]  SphPositionTargetFollAlignAxisA=+X  SphPositionTargetBaseAlignAxisA=+Y  SphPositionTargetFollAlignAxisB=+Y  SphPositionTargetBaseAlignAxisB=+Z  SphPositionTargetRotationSequenceAxes=FollowerAxes  SphPositionTargetRotationSequence=XYX  SphPositionTargetRotationSequenceAngles=[0 0 0]  SphPositionTargetRotationSequenceAnglesUnits=deg  SphPositionTargetRotationMatrix=eye(3)  SphPositionTargetSpecify=off  SphPositionTargetPriority=High  SphVelocityTargetValue=[0 0 0]  SphVelocityTargetValueUnits=deg/s  SphVelocityTargetSpecify=off  SphVelocityTargetPriority=High  SphVelocityTargetInFollowerFrame=on
  Demux2 : Demux  Outputs=12
  Mechanism Configuration : sm_lib/Utilities/Mechanism Configuration  UniformGravity=Constant  GravityVector=[0 0 -9.80665]  GravityUnits=m/s^2  LinearizationDelta=0.001
  Mux : Mux  Inputs=8
  PS-Simulink Converter1 : nesl_utility/PS-Simulink Converter  PhysicalDomain=network_engine_domain  SubClassName=ps_output  LeftPortType=input  RightPortType=output  PseudoPeriodic=off  Frequencies=[]  Unit=1  AffineConversion=off
  PS-Simulink Converter2 : nesl_utility/PS-Simulink Converter  PhysicalDomain=network_engine_domain  SubClassName=ps_output  LeftPortType=input  RightPortType=output  PseudoPeriodic=off  Frequencies=[]  Unit=1  AffineConversion=off
  Plane Offset : sm_lib/Frames and Transforms/Rigid Transform  TranslationMethod=StandardAxis  TranslationStandardOffset=height_plane/2  TranslationLengthUnit=m  TranslationStandardAxis=-Z  TranslationCartesianOffset=[0 0 0]  TranslationROffset=0  TranslationROffsetUnits=m  TranslationZOffset=0  TranslationZOffsetUnits=m  TranslationThetaOffset=0  TranslationThetaOffsetUnits=deg  RotationMethod=None  RotationAngleUnits=deg  RotationStandardAxis=+Z  RotationAngle=0.0  RotationArbitraryAxis=[0 0 1]  FollAlignAxisA=+X  BaseAlignAxisA=+Y  FollAlignAxisB=+Y  BaseAlignAxisB=+Z  RotationSequenceAxes=FollowerAxes  RotationSequence=XYX  RotationSequenceAngles=[0 0 0]  RotationSequenceAnglesUnits=deg  RotationMatrix=[1 0 0; 0 1 0; 0 0 1]
  Plane Offset1 : sm_lib/Frames and Transforms/Rigid Transform  TranslationMethod=StandardAxis  TranslationStandardOffset=height_plane/2  TranslationLengthUnit=m  TranslationStandardAxis=+Z  TranslationCartesianOffset=[0 0 0]  TranslationROffset=0  TranslationROffsetUnits=m  TranslationZOffset=0  TranslationZOffsetUnits=m  TranslationThetaOffset=0  TranslationThetaOffsetUnits=deg  RotationMethod=None  RotationAngleUnits=deg  RotationStandardAxis=+Z  RotationAngle=0.0  RotationArbitraryAxis=[0 0 1]  FollAlignAxisA=+X  BaseAlignAxisA=+Y  FollAlignAxisB=+Y  BaseAlignAxisB=+Z  RotationSequenceAxes=FollowerAxes  RotationSequence=XYX  RotationSequenceAngles=[0 0 0]  RotationSequenceAnglesUnits=deg  RotationMatrix=[1 0 0; 0 1 0; 0 0 1]
  Rate Transition : RateTransition  OutPortSampleTimeOpt=Inherit
  Rate Transition1 : RateTransition  OutPortSampleTimeOpt=Inherit
  Robot : Subsystem
  Solver Configuration : nesl_utility/Solver Configuration  PhysicalDomain=network_engine_domain  SubClassName=solver  LeftPortType=input  RightPortType=generic  Tones=[]  Harmonics=[]  SimulateNoise=off  Profile=off  UseLocalSampling=off  EnableSwitchedLinearOptims=on  FrequencyDomain=off  UseCCode=off  RelTol=0.001  AbsTol=1e-06  MinStep=1e-09  ToWorkspace=off  RevertToSquareIcSolve=off  NumHomotopyIterations=100  PhasorMode=off  PhasorModeNumHarmonics=1  DoDC=off  ResidualTolerance=1e-09  UseLocalSolver=off  LocalSolverChoice=NE_TRAPEZOIDAL_ADVANCER  LocalSolverSampleTime=0.001  DoFixedCost=off  MaxNonlinIter=3  MaxModeIter=2  LinearAlgebra=Sparse  EquationFormulation=NE_TIME_EF  DelaysMemoryBudget=1024  AutomaticFiltering=on  FilteringTimeConstant=0.001  PartitionStorageMethod=AS_NEEDED  PartitionMemoryBudget=1024  PartitionMethod=FAST
  Transform Sensor : sm_lib/Frames and Transforms/Transform Sensor  MeasurementFrame=Base  SenseAngle=off  SenseAxis=off  SenseAngle1=off  SenseAngle2=off  SenseAngle3=off  SenseQ=off  SenseR=off  SenseOmegaX=off  SenseOmegaY=off  SenseOmegaZ=off  SenseOmega1=off  SenseOmega2=off  SenseOmega3=off  SenseQDot=off  SenseRDot=off  SenseAlphaX=off  SenseAlphaY=off  SenseAlphaZ=off  SenseAlpha1=off  SenseAlpha2=off  SenseAlpha3=off  SenseQDDot=off  SenseRDDot=off  SenseX=off  SenseY=off  SenseZ=off  SenseRad=off  SenseAzim=off  SenseDist=off  SenseInc=off  SenseXDot=off  SenseYDot=off  SenseZDot=off  SenseRadDot=off  SenseAzimDot=off  SenseDistDot=off  SenseIncDot=off  SenseXDDot=on  SenseYDDot=on  SenseZDDot=off  SenseRadDDot=off  SenseAzimDDot=off  SenseDistDDot=off  SenseIncDDot=off
  World Frame : sm_lib/Frames and Transforms/World Frame
  World Frame1 : sm_lib/Frames and Transforms/World Frame
  World Plane : sm_lib/Body Elements/Solid  InertiaType=CalculateFromGeometry  Mass=1  MassUnits=kg  CenterOfMass=[0 0 0]  CenterOfMassUnits=m  MomentsOfInertia=[1 1 1]  MomentsOfInertiaUnits=kg*m^2  ProductsOfInertia=[0 0 0]  ProductsOfInertiaUnits=kg*m^2  BasedOnType=Density  Density=density  DensityUnits=kg/(m^3)  DoExposeReferenceFrame=on  SerializedFrames=<Frames/>  GraphicType=FromGeometry  MarkerShape=Sphere  MarkerSize=10  MarkerSizeUnits=m  GraphicVisPropType=SimpleVisualProperties  GraphicDiffuseColor=[1.0 1.0 0.8]  GraphicSpecularColor=[0.5 0.5 0.5 1.0]  GraphicAmbientColor=[0.15 0.15 0.15 1.0]  GraphicEmissiveColor=[0.0 0.0 0.0 1.0]  GraphicShininess=75  GraphicOpacity=0.5  GeometryShape=Brick  RectangleSize=[1 1]  RectangleSizeUnits=m  BrickDimensions="[plane_x plane_y  height_plane]"  BrickDimensionUnits=m  CylinderRadius=1  CylinderRadiusUnits=m  CylinderLength=1  CylinderLengthUnits=m  SphereRadius=1  SphereRadiusUnits=m  EllipsoidRadii=[1 1 1]  EllipsoidRadiiUnits=m  ExtrusionCrossSection=[1 1; -1 1; -1 -1; 1 -1]  ExtrusionCrossSectionUnits=m  ExtrusionLength=1  ExtrusionLengthUnits=m  PolygonNumSides=3  PolygonOuterRadius=1  PolygonOuterRadiusUnits=m  ExtGeomFileType=STL  ExtGeomFileUnits=m  RevolutionCrossSection=[1 1; 1 -1; 2 -1; 2 1]  RevolutionCrossSectionUnits=m  RevolutionExtent=Full  RevolutionAngle=180  RevolutionAngleUnits=deg
  ax : Outport
  ay : Outport  Port=2
  Fn : Outport  Port=3
  wires:
  Demux2/4 -> Robot/4(R Knee Pitch)
  q/1 -> Rate Transition/1
  Demux2/6 -> Robot/6(R Ankle Roll)
  Demux2/2 -> Robot/2(R Hip Roll)
  Demux2/11 -> Robot/11(L Ankle Pitch)
  Demux2/5 -> Robot/5(R Ankle Pitch)
  Demux2/12 -> Robot/12(L Ankle Roll)
  Demux2/1 -> Robot/1(R Hip Yaw)
  Demux2/8 -> Robot/8(L Hip Roll)
  Demux2/7 -> Robot/7(L Hip Yaw)
  Rate Transition/1 -> Demux2/1
  Demux2/3 -> Robot/3(R Hip Pitch)
  Demux2/10 -> Robot/10(L Knee Pitch)
  Demux2/9 -> Robot/9(L Hip Pitch)
  Robot/8(FnL_RearRight) -> Mux/8
  Robot/7(FnL_RearLeft) -> Mux/7
  Robot/6(FnL_FrontRight) -> Mux/6
  Robot/5(FnL_FrontLeft) -> Mux/5
  Robot/4(FnR_RearRight) -> Mux/4
  Robot/3(FnR_RearLeft) -> Mux/3
  Robot/2(FnR_FrontRight) -> Mux/2
  Robot/1(FnR_FrontLeft) -> Mux/1
  Mux/1 -> Rate Transition1/1
  Rate Transition1/1 -> Fn/1
  PS-Simulink Converter2/1 -> ay/1
  PS-Simulink Converter1/1 -> ax/1
  connections:
  Robot/RConn2 -- Transform Sensor/RConn1 -- 6-DOF Joint/RConn1
  Mechanism Configuration/RConn1 -- Solver Configuration/RConn1 -- Robot/RConn1 -- Plane Offset/LConn1 -- World Frame/RConn1
  World Plane/RConn1 -- Plane Offset1/LConn1 -- Plane Offset/RConn1
  6-DOF Joint/LConn1 -- Plane Offset1/RConn1
  World Frame1/RConn1 -- Transform Sensor/LConn1
  PS-Simulink Converter1/LConn1 -- Transform Sensor/RConn2
  PS-Simulink Converter2/LConn1 -- Transform Sensor/RConn3

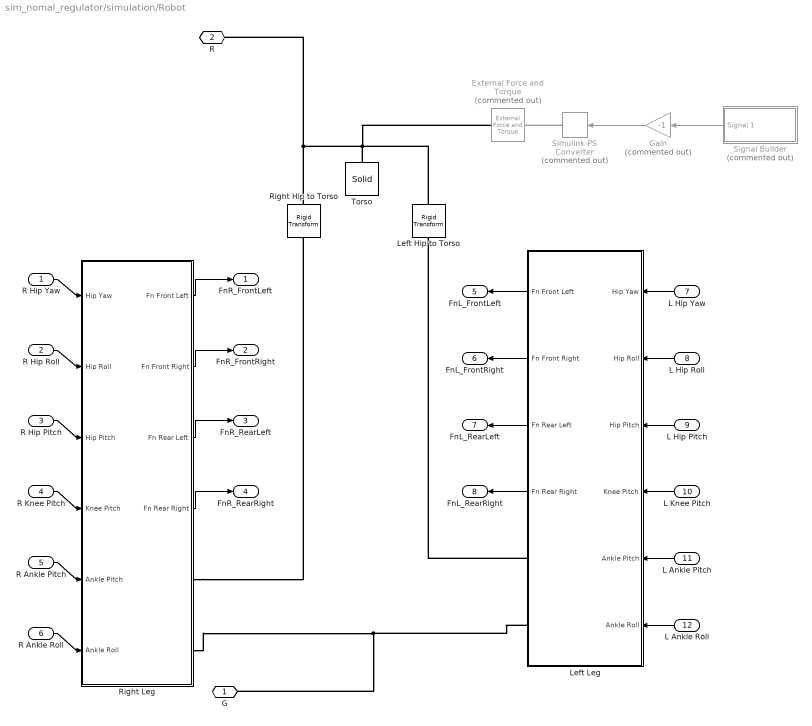
== system sim_nomal_regulator/simulation/Robot ==
  R Hip Yaw : Inport
  R Hip Roll : Inport  Port=2
  R Hip Pitch : Inport  Port=3
  R Knee Pitch : Inport  Port=4
  R Ankle Pitch : Inport  Port=5
  R Ankle Roll : Inport  Port=6
  L Hip Yaw : Inport  Port=7
  L Hip Roll : Inport  Port=8
  L Hip Pitch : Inport  Port=9
  L Knee Pitch : Inport  Port=10
  L Ankle Pitch : Inport  Port=11
  L Ankle Roll : Inport  Port=12
  External Force and Torque : sm_lib/Forces and Torques/External Force and Torque  Commented=on  ForceResolutionFrame=World  EnableForceX=on  EnableForceY=off  EnableForceZ=off  EnableForce=off  TorqueResolutionFrame=AttachedFrame  EnableTorqueX=off  EnableTorqueY=off  EnableTorqueZ=off  EnableTorque=off
  Gain : Gain  Commented=on  Gain=-1
  Left Hip to Torso : sm_lib/Frames and Transforms/Rigid Transform  TranslationMethod=Cartesian  TranslationStandardOffset=0  TranslationLengthUnit=m  TranslationStandardAxis=+Z  TranslationCartesianOffset=[torso_offset_x (torso_y/2)-0 torso_offset_z]  TranslationROffset=0  TranslationROffsetUnits=m  TranslationZOffset=0  TranslationZOffsetUnits=m  TranslationThetaOffset=0  TranslationThetaOffsetUnits=deg  RotationMethod=None  RotationAngleUnits=deg  RotationStandardAxis=+Z  RotationAngle=0.0  RotationArbitraryAxis=[0 0 1]  FollAlignAxisA=+X  BaseAlignAxisA=+Y  FollAlignAxisB=+Y  BaseAlignAxisB=+Z  RotationSequenceAxes=FollowerAxes  RotationSequence=XYX  RotationSequenceAngles=[0 0 0]  RotationSequenceAnglesUnits=deg  RotationMatrix=[1 0 0; 0 1 0; 0 0 1]
  Left Leg : Subsystem
  Right Hip to Torso : sm_lib/Frames and Transforms/Rigid Transform  TranslationMethod=Cartesian  TranslationStandardOffset=0  TranslationLengthUnit=m  TranslationStandardAxis=+Z  TranslationCartesianOffset=[torso_offset_x (-torso_y/2)+0 torso_offset_z]  TranslationROffset=0  TranslationROffsetUnits=m  TranslationZOffset=0  TranslationZOffsetUnits=m  TranslationThetaOffset=0  TranslationThetaOffsetUnits=deg  RotationMethod=None  RotationAngleUnits=deg  RotationStandardAxis=+Z  RotationAngle=0.0  RotationArbitraryAxis=[0 0 1]  FollAlignAxisA=+X  BaseAlignAxisA=+Y  FollAlignAxisB=+Y  BaseAlignAxisB=+Z  RotationSequenceAxes=FollowerAxes  RotationSequence=XYX  RotationSequenceAngles=[0 0 0]  RotationSequenceAnglesUnits=deg  RotationMatrix=[1 0 0; 0 1 0; 0 0 1]
  Right Leg : Subsystem
  Signal Builder : Subsystem  Tag=STV Subsys  Commented=on  LoadFcn=sigbuilder_block('load');  StartFcn=sigbuilder_block('start');  StopFcn=sigbuilder_block('stop');  ClipboardFcn=sigbuilder_block('clipboard');  mask(Sigbuilder block){tuvar=[0:10]}
      mask help: Simulink:masks:SigbuilderBlock_MD
      mask init:
      | if ~strcmp(get_param(bdroot(gcbh),'SimulationStatus'),'stopped') tuvar = sigbuilder_block('maskInit'); end
      settings: CopyFcn=sigbuilder_block('copy');  DeleteFcn=sigbuilder_block('delete');  ModelCloseFcn=sigbuilder_block('modelClose');  PreSaveFcn=sigbuilder_block('preSave');  PauseFcn=sigbuilder_block('pause');  ContinueFcn=sigbuilder_block('continue');  NameChangeFcn=sigbuilder_block('namechange');  OpenFcn=sigbuilder_block('open',[437.6 199.2 550.4 400 ]);  CloseFcn=sigbuilder_block('close');
      mask Display: plot(0, 0, 100, 100,[2, 2, 32, 32, 2], [68, 8, 8, 68, 68],[32, 2], [38, 38], [32, 19, 2],[53, 60, 44], [32, 17, 17, 2],[16, 16, 31, 31]);txt = getActiveGroup(gcbh);text(2, 100, txt,'verticalAlignment', 'top');
  Simulink-PS Converter : nesl_utility/Simulink-PS Converter  Commented=on  PhysicalDomain=network_engine_domain  SubClassName=ps_input  LeftPortType=input  RightPortType=output  PseudoPeriodic=off  Frequencies=[]  NoiseDistribution=none  NoiseParameters=[]  Unit=N  AffineConversion=off  FilteringAndDerivatives=provide  SimscapeFilterOrder=1  InputFilterTimeConstant=0.001  UdotUserProvided=0
  Torso : sm_lib/Body Elements/Solid  InertiaType=PointMass  Mass=0.323  MassUnits=kg  CenterOfMass=[0 0 0]  CenterOfMassUnits=m  MomentsOfInertia=[1 1 1]  MomentsOfInertiaUnits=kg*m^2  ProductsOfInertia=[1 1 1]  ProductsOfInertiaUnits=kg*m^2  BasedOnType=Density  Density=density  DensityUnits=kg/m^3  DoExposeReferenceFrame=on  SerializedFrames=<Frames/>  GraphicType=FromGeometry  MarkerShape=Sphere  MarkerSize=10  GraphicVisPropType=SimpleVisualProperties  GraphicDiffuseColor=[0.5 0.5 0.5]  GraphicSpecularColor=[0.5 0.5 0.5 1.0]  GraphicAmbientColor=[0.15 0.15 0.15 1.0]  GraphicEmissiveColor=[0.0 0.0 0.0 1.0]  GraphicShininess=75  GraphicOpacity=1.0  GeometryShape=Brick  RectangleSize=[1 1]  RectangleSizeUnits=m  BrickDimensions=[torso_x torso_y torso_z]  BrickDimensionUnits=m  CylinderRadius=1  CylinderRadiusUnits=m  CylinderLength=1  CylinderLengthUnits=m  SphereRadius=1  SphereRadiusUnits=m  EllipsoidRadii=[1 1 1]  EllipsoidRadiiUnits=m  ExtrusionCrossSection=[1 1; -1 1; -1 -1; 1 -1]  ExtrusionCrossSectionUnits=m  ExtrusionLength=1  ExtrusionLengthUnits=m  PolygonNumSides=3  PolygonOuterRadius=1  PolygonOuterRadiusUnits=m  ExtGeomFileType=STEP  ExtGeomFileUnits=m  RevolutionCrossSection=[1 1; 1 -1; 2 -1; 2 1]  RevolutionCrossSectionUnits=m  RevolutionExtent=Full  RevolutionAngle=180  RevolutionAngleUnits=deg
  G : PMIOPort  Side=Right
  R : PMIOPort  Port=2  Side=Right
  FnR_FrontLeft : Outport
  FnR_FrontRight : Outport  Port=2
  FnR_RearLeft : Outport  Port=3
  FnR_RearRight : Outport  Port=4
  FnL_FrontLeft : Outport  Port=5
  FnL_FrontRight : Outport  Port=6
  FnL_RearLeft : Outport  Port=7
  FnL_RearRight : Outport  Port=8
  wires:
  R Hip Pitch/1 -> Right Leg/3(Hip Pitch)
  R Ankle Roll/1 -> Right Leg/6(Ankle Roll)
  R Ankle Pitch/1 -> Right Leg/5(Ankle Pitch)
  R Hip Roll/1 -> Right Leg/2(Hip Roll)
  R Knee Pitch/1 -> Right Leg/4(Knee Pitch)
  R Hip Yaw/1 -> Right Leg/1(Hip Yaw)
  L Hip Yaw/1 -> Left Leg/1(Hip Yaw)
  L Ankle Roll/1 -> Left Leg/6(Ankle Roll)
  L Hip Roll/1 -> Left Leg/2(Hip Roll)
  L Hip Pitch/1 -> Left Leg/3(Hip Pitch)
  L Ankle Pitch/1 -> Left Leg/5(Ankle Pitch)
  L Knee Pitch/1 -> Left Leg/4(Knee Pitch)
  Signal Builder/1(Signal 1) -> Gain/1
  Right Leg/1(Fn Front Left) -> FnR_FrontLeft/1
  Right Leg/2(Fn Front Right) -> FnR_FrontRight/1
  Right Leg/3(Fn Rear Left) -> FnR_RearLeft/1
  Right Leg/4(Fn Rear Right) -> FnR_RearRight/1
  Left Leg/1(Fn Front Left) -> FnL_FrontLeft/1
  Left Leg/3(Fn Rear Left) -> FnL_RearLeft/1
  Left Leg/2(Fn Front Right) -> FnL_FrontRight/1
  Left Leg/4(Fn Rear Right) -> FnL_RearRight/1
  Gain/1 -> Simulink-PS Converter/1
  connections:
  Left Leg/RConn1 -- Left Hip to Torso/RConn1
  Right Leg/RConn1 -- Right Hip to Torso/RConn1
  Torso/RConn1 -- External Force and Torque/RConn1 -- Left Hip to Torso/LConn1 -- R/RConn1 -- Right Hip to Torso/LConn1
  Right Leg/RConn2 -- Left Leg/RConn2 -- G/RConn1
  Simulink-PS Converter/RConn1 -- External Force and Torque/LConn1
